simulink model "wind_power_plant"  (R2022b)
settings: Solver=VariableStepAuto  StartTime=0.0  StopTime=30.0  RelTol=1e-3
libraries: spsGroundLib x2, spsSeriesRLCBranchLib x1, spsThreePhaseProgrammableVoltageSourceLib x1, spsThreePhaseSeriesRLCLoadLib x1, spsThreePhaseTransformerInductanceMatrixTypeTwoWindingsLib x1, spsWindTurbineInductionGeneratorPhasorTypeLib x1, spspowerguiLib x1
settings Model: Creator=Haina Bhawnani  LastModifiedBy=Haina Bhawnani

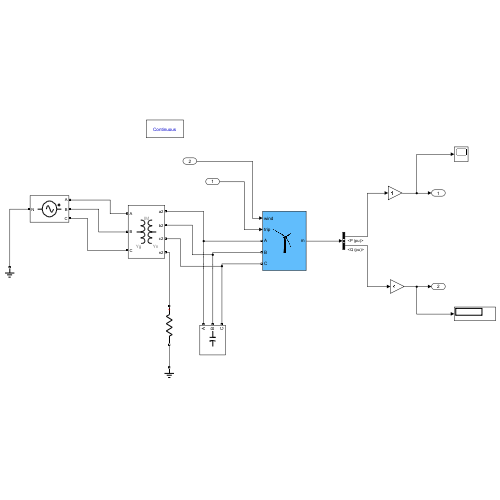
[thumbnail: Simulink's stored preview of the top-level diagram]
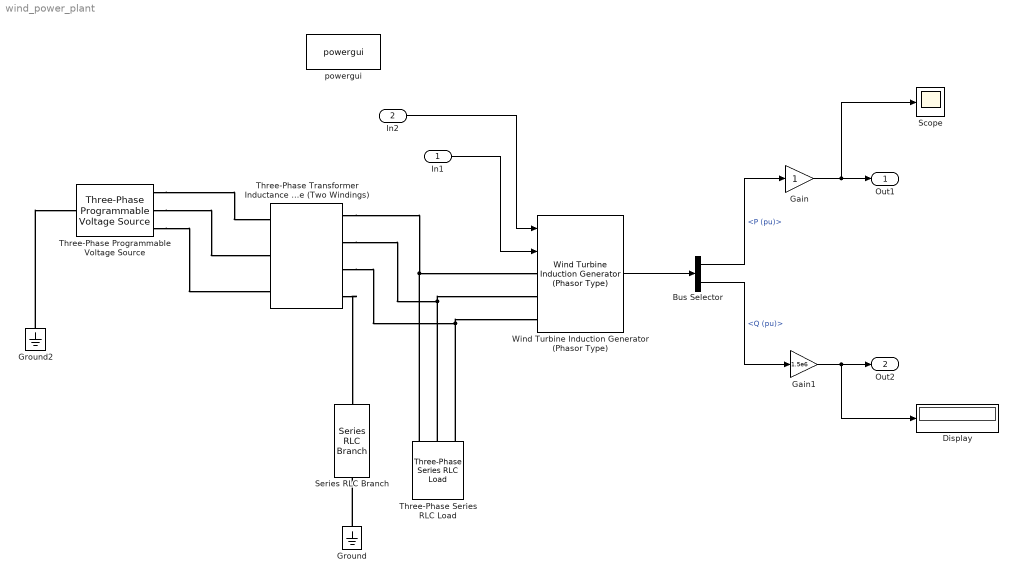
== system wind_power_plant ==
  In1 : Inport
  In2 : Inport  Port=2
  Bus Selector : BusSelector  OutputSignals=P (pu),Q (pu)
  Display : Display
  Gain : Gain
  Gain1 : Gain  Gain=1.5e6
  Ground : spsGroundLib/Ground  LConnTagsString=a
  Ground2 : spsGroundLib/Ground  LConnTagsString=a
  Scope : Scope
  Series RLC Branch : spsSeriesRLCBranchLib/Series RLC Branch  LConnTagsString=__new0  RConnTagsString=__new0  BranchType=R  Resistance=66  Inductance=1e-3  SetiL0=off  InitialCurrent=0  Capacitance=1e-6  Setx0=off  InitialVoltage=0  Measurements=None
  Three-Phase Programmable Voltage Source : spsThreePhaseProgrammableVoltageSourceLib/Three-Phase Programmable Voltage Source  PositiveSequence="[25e3  0 60]"  VariationEntity=None  VariationType=Table of time-amplitude pairs  VariationTypeAlt=Step  VariationStep=0.5  VariationRate=10  VariationMagnitude=0.3  VariationFrequency=2  VariationTiming=[1 2]  VariationPhaseA=off  Amplitudes=[1 0.8 1.2 1.0]  TimeValues=[0 0.1 0.15 0.2]  HarmonicGeneration=off  HarmonicA=[3 0.2 -25 0]  HarmonicB=[2 0.15 35 2]  Timing="[0.05  3]"  BusType=swing  Pref=0  Qref=0  Qmin=-inf  Qmax=inf
  Three-Phase Series RLC Load : spsThreePhaseSeriesRLCLoadLib/Three-Phase Series RLC Load  LConnTagsString=A|B|C  Configuration=Delta  NominalVoltage=575  Vabc=[1e3 1e3 1e3]  Vabcp=[1e3 1e3 1e3]  NominalFrequency=60  UnbalancedPower=off  ActivePower=0  InductivePower=0  CapacitivePower=400e3  Pabc=[10e3 9e3 11e3]  QLabc=[100 90 110]  QCabc=[100 90 110]  Pabcp=[10e3 9e3 11e3]  QLabcp=[100 90 110]  QCabcp=[100 90 110]  Measurements=None  LoadType=constant Z
  Three-Phase Transformer Inductance Matrix Type (Two Windings) : spsThreePhaseTransformerInductanceMatrixTypeTwoWindingsLib/Three-Phase Transformer Inductance Matrix Type (Two Windings)  CoreType=Three-limb or five-limb core  Winding1Connection=Yg  Winding2Connection=Yn  AutoTransformer=off  Measurements=None  NominalPower=[4e6, 60]  VLLnom=[25e3, 575]  WindingResistances=[0.025/30, 0.025/30]  NoLoadIexcPos=2  NoLoadPlossPos=1000  ShortCircuitReactancePos=0.06  ShortCircuitReactancePosAuto=0.06  NoLoadIexcZero=100  NoLoadPlossZero=1500  ShortCircuitReactanceZero=0.03  ShortCircuitReactanceZeroAuto=0.03
      settings: LibrarySourceBlock=|
      | sps_lib/Power Grid Elements/Three-Phase Transformer
      | Inductance Matrix Type
      | (Two Windings)
  Wind Turbine Induction Generator (Phasor Type) : spsWindTurbineInductionGeneratorPhasorTypeLib/Wind Turbine Induction Generator (Phasor Type)  ExternalTm=off  nom=[1.5e6/0.9, 575, 60]  sta=[ 0.004843, 0.1248]  rot=[ 0.004377, 0.1791]  Lm=6.77  mec=[5.04, 0.01, 3]  init="[ -0.01,0,   0,0,0,   0,0,0 ]"  pitch_angle=0  Pmec=1.5e6  wind_base=9  speed_nom=1  P_wind_base=1  K_pitch_gain=[5 25]  pitch_max=45  pitch_rate=2
      settings: LibrarySourceBlock=|
      | sps_lib/Electrical Machines/Wind Turbine
      | Induction Generator
      | (Phasor Type)
  powergui : spspowerguiLib/powergui  Priority=1  SimulationMode=Continuous  SampleTime=50e-6  frequency=60  Iterations=50  frequencyindice=60  Pbase=100e6  ErrMax=1e-4  UnitsV=kV  UnitsW=MW  buscounter=0  FunctionMessages=off  echomessages=off  EnableUseOfTLC=off  CurrentSourceSwitches=off  DisableSnubberDevices=off  DisableRonSwitches=off  DisableVfSwitches=off  DisplayEquations=off  AutomaticDiscreteSolvers=off  SolverType=Tustin/Backward Euler (TBE)  Interpol=off  ExternalGateDelay=off  methode=off  Ts=100  x0status=blocks  SPID=on  SwTol=0  HookPort=off  NonlinearTolerance=1e-4  nMaxIteration=100  ContinueOnMaxIteration=off  RestoreLinks=warning  ResistiveCurrentMeasurement=off  Frange=[0:2:500]  Ylog=off  Xlog=on  ShowGrid=off  save=off  variable=ZData  structure=0  ZoomFFT=off  StartTime=0.0  cycles=1  DisplayStyle=1  fundamental=60  FreqAxis=off  MaxFrequency=1000  frequencyindicesteady=1  RmsSteady=1  display=off
  Out1 : Outport
  Out2 : Outport  Port=2
  wires:
  Wind Turbine Induction Generator (Phasor Type)/1 -> Bus Selector/1
  Bus Selector/1 -> Gain/1  "<P (pu)>"
  Bus Selector/2 -> Gain1/1  "<Q (pu)>"
  Gain/1 -> Scope/1, Out1/1
  Gain1/1 -> Display/1, Out2/1
  In1/1 -> Wind Turbine Induction Generator (Phasor Type)/2
  In2/1 -> Wind Turbine Induction Generator (Phasor Type)/1
  connections:
  Ground/LConn1 -- Series RLC Branch/RConn1
  Three-Phase Transformer Inductance Matrix Type (Two Windings)/RConn1 -- Three-Phase Series RLC Load/LConn1 -- Wind Turbine Induction Generator (Phasor Type)/LConn1
  Three-Phase Transformer Inductance Matrix Type (Two Windings)/RConn2 -- Three-Phase Series RLC Load/LConn2 -- Wind Turbine Induction Generator (Phasor Type)/LConn2
  Three-Phase Transformer Inductance Matrix Type (Two Windings)/RConn4 -- Series RLC Branch/LConn1
  Three-Phase Transformer Inductance Matrix Type (Two Windings)/RConn3 -- Three-Phase Series RLC Load/LConn3 -- Wind Turbine Induction Generator (Phasor Type)/LConn3
  Three-Phase Programmable Voltage Source/RConn1 -- Three-Phase Transformer Inductance Matrix Type (Two Windings)/LConn1
  Three-Phase Programmable Voltage Source/RConn2 -- Three-Phase Transformer Inductance Matrix Type (Two Windings)/LConn2
  Three-Phase Programmable Voltage Source/RConn3 -- Three-Phase Transformer Inductance Matrix Type (Two Windings)/LConn3
  Ground2/LConn1 -- Three-Phase Programmable Voltage Source/LConn1
